simulink model "CarAccelerator"  (R2023a)
settings: Solver=FixedStepAuto  StartTime=0.0  StopTime=4  FixedStep=0.25  RelTol=1e-3
libraries: simulink x3
settings Model: Creator=Alielden  LastModifiedBy=Alielden

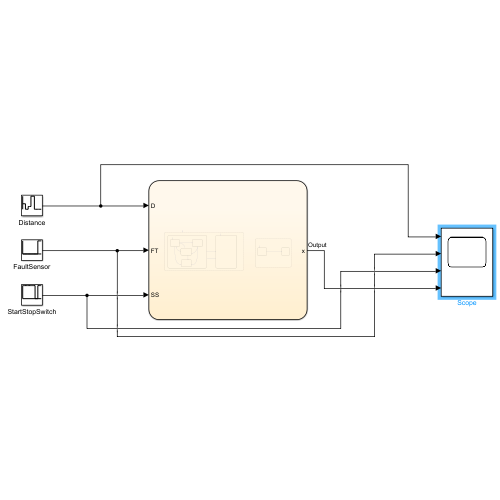
[thumbnail: Simulink's stored preview of the top-level diagram]
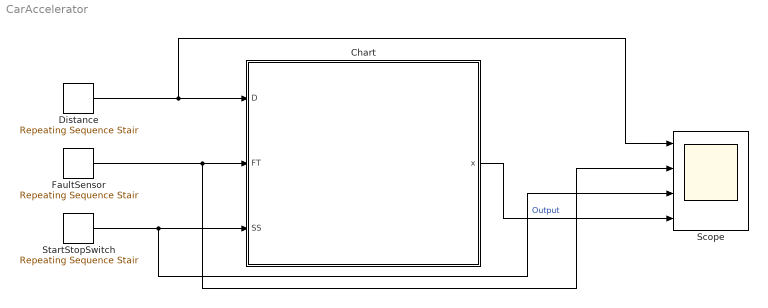
== system CarAccelerator ==
  Chart : Stateflow chart  TreatAsAtomicUnit=on
  Distance : simulink/Sources/Repeating Sequence Stair  OutValues="[6 6 4 4 5 5 9 9 4 4 4 4 4  ].'"  tsamp=-1  OutMin=[]  OutMax=[]  OutDataTypeStr=double  OutputDataTypeScalingMode=double  OutDataType=fixdt(0,8)  ConRadixGroup=Best Precision: Vector-wise  OutScaling=2^-12
  FaultSensor : simulink/Sources/Repeating Sequence Stair  OutValues=[0 0 0 0 0 0 0 0 0 0 0 0 1 1 1].'  tsamp=-1  OutMin=[]  OutMax=[]  OutDataTypeStr=double  OutputDataTypeScalingMode=double  OutDataType=fixdt(0,8)  ConRadixGroup=Best Precision: Vector-wise  OutScaling=2^-12
  Scope : Scope  NumInputPorts=4
  StartStopSwitch : simulink/Sources/Repeating Sequence Stair  OutValues=[1 1 1 1 1 1 1 1 1 1 0 0 1 1 1].'  tsamp=-1  OutMin=[]  OutMax=[]  OutDataTypeStr=double  OutputDataTypeScalingMode=double  OutDataType=fixdt(0,8)  ConRadixGroup=Best Precision: Vector-wise  OutScaling=2^-12
  wires:
  StartStopSwitch/1 -> Scope/3, Chart/3(SS)
  FaultSensor/1 -> Scope/2, Chart/2(FT)
  Distance/1 -> Scope/1, Chart/1(D)
  Chart/1(x) -> Scope/4  "Output"

== stateflow chart CarAccelerator/Chart ==
  note: x=1 acc
      | x=-1 de_acc
      | x=0 = nothing
      | x=-2 stop
      | x=-3 error
  state Regular_System [parallel]
    settings: executionOrder=1
    state On_State
      state Accelerate
        en:
        x=1;
      state DeAccelerate
        en:
        x=-1;
      state Nothing
        en:
        x=0;
      state Stop
        en:
        x=-2;
      (default) -> Accelerate
      Accelerate -> DeAccelerate [order 1] : [D<5]
      Accelerate -> Nothing [order 3] : [D==5]
      Accelerate -> Stop [order 2] : [D<2]
      Nothing -> Accelerate [order 1] : [D>8]
      DeAccelerate -> Stop [order 2] : [D<2]
      DeAccelerate -> Nothing [order 1] : [D==5]
      Nothing -> Stop [order 2] : [D<2]
    state Off_State
      en:
      x=-2;
    (default) -> Off_State
    On_State -> Off_State : [SS==0]
    Off_State -> On_State : [SS==1]
  state Fault_Detection [parallel]
    settings: executionOrder=2
    state Fault
      en:
      x=-3;
    state InitialFault
    (default) -> InitialFault
    InitialFault -> Fault : [FT==1]
  (default) -> Regular_System
  data: D input; FT input; x output; SS input
